simulink model "sim05"  (R2022b)
settings: Solver=ode4  StartTime=0.0  StopTime=inf  FixedStep=0.001  RelTol=1e-3
undefined symbols (not defined in the file or in its folder): National_Instruments, PCI
libraries: sldrtlib x3, cstblocks x1
settings Model: SimulationMode=external  ExtModeTrigDuration=60000  ExtModeArchiveMode=auto  ExtModeArchiveFileName=data  ExtModeArchiveDirName=E:\work\me-clab2\Lab05  ExtModeAddSuffixToVar=on  Creator=me-clab2  LastModifiedBy=X1
settings SolverCC: AlgebraicLoopSolver=TrustRegion
settings DebuggingCC: UnconnectedInputMsg=warning  UnconnectedOutputMsg=warning  UnconnectedLineMsg=warning  SFMachineParentedDataDiag=warning
settings ModelReferenceCC: EnableRefExpFcnMdlSchedulingChecks=on
settings RTWCC: Description=Simulink Desktop Real-Time  SystemTargetFile=sldrt.tlc  TemplateMakefile=sldrt.tmf  RTWCompilerOptimization=on
settings CodeAppCC: MaxIdLength=95
settings SimulinkDesktopRealTimeCC: TargetPreCompLibLocation=C:\Program Files\MATLAB\R2020a\toolbox\sldrt\lib\win64

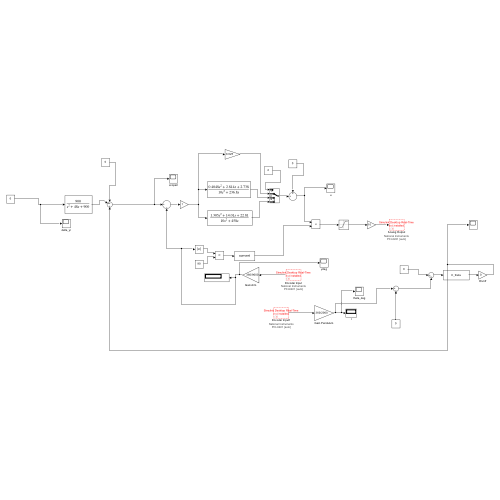
[thumbnail: Simulink's stored preview of the top-level diagram]
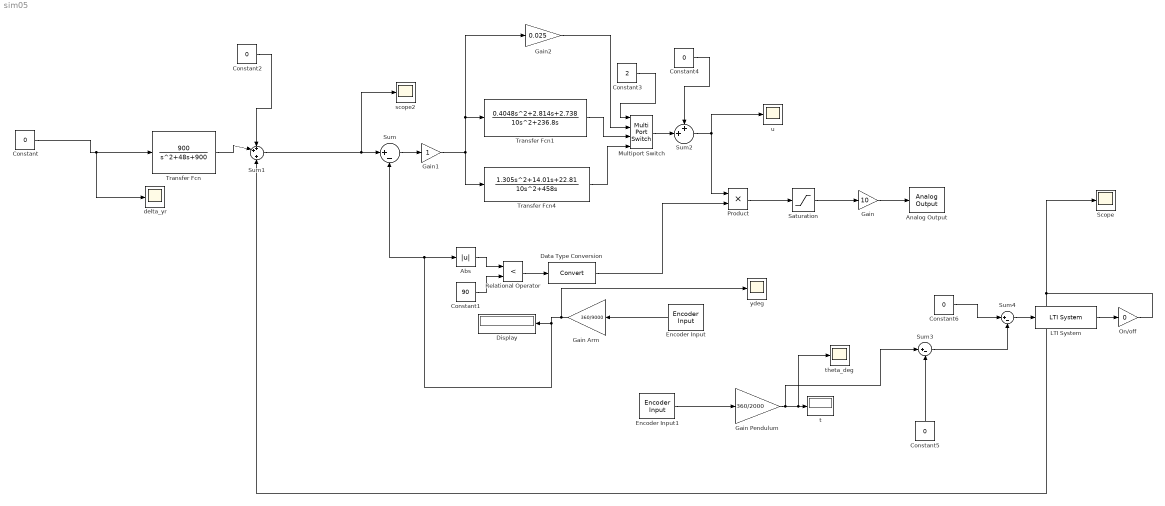
== system sim05 ==
  Abs : Abs  SaturateOnIntegerOverflow=off
  Analog Output : sldrtlib/Analog Output  SampleTime=0.001  MaxMissedTicks=10  ShowMissedTicks=off  YieldWhenWaiting=off  DrvName=National_Instruments/PCI-6221  DrvAddress=4294967295  DrvOptions=[0 0 0 2 2]  Channels=[2]  RangeMode=1  VoltRange=1  InitialValue=0  FinalValue=0
      settings: AttributesFormatString=National Instruments\nPCI-6221 [auto]
  Constant{,2,4..6} (5 alike) : Constant  Value=0
  Constant1 : Constant  Value=90
  Constant3 : Constant  Value=2
  Data Type Conversion : DataTypeConversion  SaturateOnIntegerOverflow=off  RndMeth=Floor
  Display : Display
  Encoder Input : sldrtlib/Encoder Input  SampleTime=0.001  MaxMissedTicks=10  ShowMissedTicks=off  YieldWhenWaiting=off  DrvName=National_Instruments/PCI-6221  DrvAddress=4294967295  DrvOptions=[0 0 0 2 2]  Channels=[1]  QuadMode=3  IndexPulse=1  InputFilter=Inf  DataType=1
      settings: AttributesFormatString=National Instruments\nPCI-6221 [auto]
  Encoder Input1 : sldrtlib/Encoder Input  SampleTime=0.001  MaxMissedTicks=10  ShowMissedTicks=off  YieldWhenWaiting=off  DrvName=National_Instruments/PCI-6221  DrvAddress=4294967295  DrvOptions=[0 0 0 2 2]  Channels=[2]  QuadMode=3  IndexPulse=1  InputFilter=Inf  DataType=1
      settings: AttributesFormatString=National Instruments\nPCI-6221 [auto]
  Gain : Gain  Gain=10
  Gain Arm : Gain  Gain=360/9000
  Gain Pendulum : Gain  Gain=360/2000
  Gain1 : Gain
  Gain2 : Gain  Gain=0.025
  LTI System : cstblocks/LTI System  sys=C_theta  IC=[]
  Multiport Switch : MultiPortSwitch  SaturateOnIntegerOverflow=off  InputSameDT=off
  On/off : Gain  Gain=0
  Product : Product
  Relational Operator : RelationalOperator  Operator=<  OutDataTypeStr=boolean  RndMeth=Simplest  InputSameDT=off
  Saturation : Saturate  UpperLimit=1  LowerLimit=-1
  Scope : Scope
  Sum : Sum  Inputs=|+-
  Sum1 : Sum  Inputs=++|+
  Sum2 : Sum  Inputs=++|
  Sum3 : Sum  Inputs=|+-
  Sum4 : Sum  Inputs=|+-
  Transfer Fcn : TransferFcn  Numerator=[900]  Denominator=[1 48 900]
  Transfer Fcn1 : TransferFcn  Numerator=[0.4048 2.814 2.738]  Denominator=[10 236.8 0]
  Transfer Fcn4 : TransferFcn  Numerator=[1.305 14.01 22.81]  Denominator=[10 458 0]
  delta_yr : Scope
  scope2 : Scope
  t : Display
  theta_deg : Scope
  u : Scope
  ydeg : Scope
  wires:
  Encoder Input/1 -> Gain Arm/1
  Gain Arm/1 -> ydeg/1, Display/1, Abs/1, Sum/2
  Saturation/1 -> Gain/1
  Gain/1 -> Analog Output/1
  Sum/1 -> Gain1/1
  Gain1/1 -> Gain2/1, Transfer Fcn1/1, Transfer Fcn4/1
  Product/1 -> Saturation/1
  Abs/1 -> Relational Operator/1
  Constant1/1 -> Relational Operator/2
  Relational Operator/1 -> Data Type Conversion/1
  Data Type Conversion/1 -> Product/2
  Transfer Fcn/1 -> Sum1/2
  Sum1/1 -> scope2/1, Sum/1
  Constant2/1 -> Sum1/1
  Gain2/1 -> Multiport Switch/2
  Transfer Fcn1/1 -> Multiport Switch/3
  Transfer Fcn4/1 -> Multiport Switch/4
  Constant3/1 -> Multiport Switch/1
  Multiport Switch/1 -> Sum2/2
  Sum2/1 -> Product/1, u/1
  Constant4/1 -> Sum2/1
  Encoder Input1/1 -> Gain Pendulum/1
  Gain Pendulum/1 -> Sum3/1, theta_deg/1, t/1
  Constant5/1 -> Sum3/2
  Sum3/1 -> Sum4/2
  Constant6/1 -> Sum4/1
  Sum4/1 -> LTI System/1
  LTI System/1 -> On/off/1
  On/off/1 -> Scope/1, Sum1/3
  Constant/1 -> delta_yr/1, Transfer Fcn/1
